simulink model "kinematic_controller_system"  (R2014b)
settings: Solver=ode3  StartTime=0.0  StopTime=tfinal  FixedStep=Tsample  RelTol=1e-3
libraries: DiffSteer_model x2, Controllers x2
settings Model: Creator=Felipe  LastModifiedBy=Martins
settings DataIOCC: LimitDataPoints=off
settings DebuggingCC: UnderspecifiedInitializationDetection=Classic  MergeDetectMultiDrivingBlocksExec=none  SolverPrmCheckMsg=none  StateNameClashWarn=warning

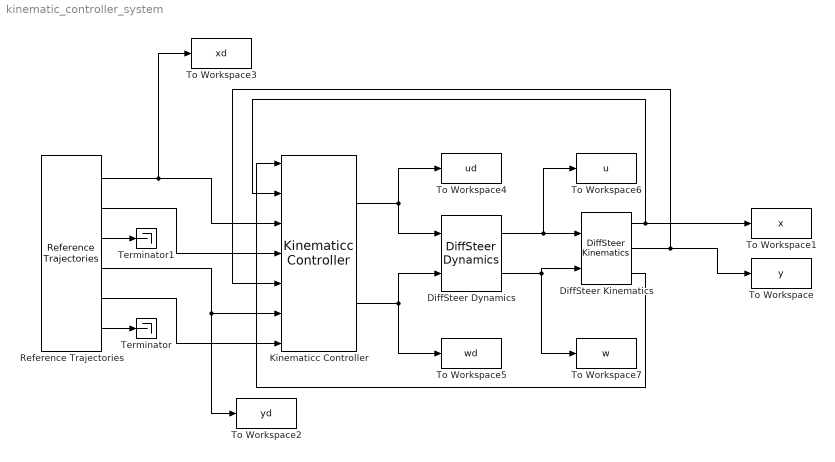
== system kinematic_controller_system ==
  DiffSteer Dynamics : DiffSteer_model/DiffSteer Dynamics  umax=0.75  wmax=1.745  dumax=0.3  dwmax=1.745  param=[0.2604 0.2509 -0.000499 0.9965 0.00263 1.0768]
  DiffSteer Kinematics : DiffSteer_model/DiffSteer Kinematics  x0=[0.2, 0, 0]  a=0.2  umax=0.75  wmax=1.745  dumax=0.3  dwmax=1.745
  Kinematicc Controller : Controllers/Kinematicc Controller  kx=0.1  ky=0.1  lx=0.1  ly=0.1  a=0.2
  Reference Trajectories : Controllers/Reference Trajectories  trajectory_type=2  wf=0.25  raio_ref_1=1  delta_raio=-0.1  t_delta_raio=60  xd=[1, -2.5]
  Terminator : Terminator
  Terminator1 : Terminator
  To Workspace : ToWorkspace  VariableName=y  SampleTime=-1
  To Workspace1 : ToWorkspace  VariableName=x  SampleTime=-1
  To Workspace2 : ToWorkspace  VariableName=yd  SampleTime=-1
  To Workspace3 : ToWorkspace  VariableName=xd  SampleTime=-1
  To Workspace4 : ToWorkspace  VariableName=ud  SampleTime=-1
  To Workspace5 : ToWorkspace  VariableName=wd  SampleTime=-1
  To Workspace6 : ToWorkspace  VariableName=u  SampleTime=-1
  To Workspace7 : ToWorkspace  VariableName=w  SampleTime=-1
  wires:
  Reference Trajectories/1 -> To Workspace3/1, Kinematicc Controller/3
  Reference Trajectories/2 -> Kinematicc Controller/4
  Reference Trajectories/4 -> To Workspace2/1, Kinematicc Controller/6
  Reference Trajectories/5 -> Kinematicc Controller/7
  DiffSteer Kinematics/1 -> Kinematicc Controller/2, To Workspace1/1
  DiffSteer Kinematics/2 -> To Workspace/1, Kinematicc Controller/5
  DiffSteer Kinematics/3 -> Kinematicc Controller/1
  Kinematicc Controller/1 -> DiffSteer Dynamics/1, To Workspace4/1
  Kinematicc Controller/2 -> To Workspace5/1, DiffSteer Dynamics/2
  DiffSteer Dynamics/1 -> To Workspace6/1, DiffSteer Kinematics/1
  DiffSteer Dynamics/2 -> DiffSteer Kinematics/2, To Workspace7/1
  Reference Trajectories/3 -> Terminator1/1
  Reference Trajectories/6 -> Terminator/1
